simulink model "EiTR2018B (1)"  (R2019b)
settings: Solver=VariableStepAuto  StartTime=0.0  StopTime=600  RelTol=1e-3
values from neighbouring files (symbols this model uses):
  boardingTime = 15    [configFile.m]
  transportTime = 60    [configFile.m]
undefined symbols (not defined in the file or in its folder): m, n
(part 2 of 2)

== stateflow chart EiTR2018B (1)/Person generator two ==
  settings: enableNonTerminalStates=1
  state Hour_24
    state min_0
      state IDLE
        entry:
        lambda = 4;
        dt =60* rand();
        Persons.data=poissrnd(lambda);
      state Wait
      (default) -> Hour_24.min_0.IDLE
      Hour_24.min_0.Wait -> Hour_24.min_0.IDLE : after(dt,sec){send(Persons)}
      Hour_24.min_0.IDLE -> Hour_24.min_0.Wait
    state min_45
      state IDLE
        entry:
        lambda = 4;
        dt =60* rand();
        Persons.data=poissrnd(lambda);
      state Wait
      (default) -> Hour_24.min_45.IDLE : {dt=0;}
      Hour_24.min_45.Wait -> Hour_24.min_45.IDLE : after(dt,sec){send(Persons)}
      Hour_24.min_45.IDLE -> Hour_24.min_45.Wait
    state min_15
      state IDLE
        entry:
        lambda = 4;
        dt =60* rand();
        Persons.data=poissrnd(lambda);
      state Wait
      (default) -> Hour_24.min_15.IDLE : {dt=0;}
      Hour_24.min_15.Wait -> Hour_24.min_15.IDLE : after(dt,sec){send(Persons)}
      Hour_24.min_15.IDLE -> Hour_24.min_15.Wait
    state min_30
      state IDLE
        entry:
        lambda = 4;
        dt =60* rand();
        Persons.data=poissrnd(lambda);
      state Wait
      (default) -> Hour_24.min_30.IDLE : {dt=0;}
      Hour_24.min_30.Wait -> Hour_24.min_30.IDLE : after(dt,sec){send(Persons)}
      Hour_24.min_30.IDLE -> Hour_24.min_30.Wait
    (default) -> Hour_24.min_0
    Hour_24.min_0 -> Hour_24.min_15 : after(60*15,sec)
    Hour_24.min_30 -> Hour_24.min_45 : after(60*15,sec)
    Hour_24.min_15 -> Hour_24.min_30 : after(60*15,sec)
  state Hour_23
    state min_0
      state IDLE
        entry:
        lambda = 4;
        dt =60* rand();
        Persons.data=poissrnd(lambda);
      state Wait
      (default) -> Hour_23.min_0.IDLE
      Hour_23.min_0.Wait -> Hour_23.min_0.IDLE : after(dt,sec){send(Persons)}
      Hour_23.min_0.IDLE -> Hour_23.min_0.Wait
    state min_45
      state IDLE
        entry:
        lambda = 4;
        dt =60* rand();
        Persons.data=poissrnd(lambda);
      state Wait
      (default) -> Hour_23.min_45.IDLE : {dt=0;}
      Hour_23.min_45.Wait -> Hour_23.min_45.IDLE : after(dt,sec){send(Persons)}
      Hour_23.min_45.IDLE -> Hour_23.min_45.Wait
    state min_15
      state IDLE
        entry:
        lambda = 4;
        dt =60* rand();
        Persons.data=poissrnd(lambda);
      state Wait
      (default) -> Hour_23.min_15.IDLE : {dt=0;}
      Hour_23.min_15.Wait -> Hour_23.min_15.IDLE : after(dt,sec){send(Persons)}
      Hour_23.min_15.IDLE -> Hour_23.min_15.Wait
    state min_30
      state IDLE
        entry:
        lambda = 4;
        dt =60* rand();
        Persons.data=poissrnd(lambda);
      state Wait
      (default) -> Hour_23.min_30.IDLE : {dt=0;}
      Hour_23.min_30.Wait -> Hour_23.min_30.IDLE : after(dt,sec){send(Persons)}
      Hour_23.min_30.IDLE -> Hour_23.min_30.Wait
    (default) -> Hour_23.min_0
    Hour_23.min_0 -> Hour_23.min_15 : after(60*15,sec)
    Hour_23.min_30 -> Hour_23.min_45 : after(60*15,sec)
    Hour_23.min_15 -> Hour_23.min_30 : after(60*15,sec)
  state Hour_1
    state min_0
      state IDLE
        entry:
        lambda = 0.5;
        dt =60* rand();
        Persons.data=poissrnd(lambda);
      state Wait
      (default) -> Hour_1.min_0.IDLE
      Hour_1.min_0.Wait -> Hour_1.min_0.IDLE : after(dt,sec){send(Persons)}
      Hour_1.min_0.IDLE -> Hour_1.min_0.Wait
    state min_45
      state IDLE
        entry:
        lambda = 4;
        dt =60* rand();
        Persons.data=poissrnd(lambda);
      state Wait
      (default) -> Hour_1.min_45.IDLE : {dt=0;}
      Hour_1.min_45.Wait -> Hour_1.min_45.IDLE : after(dt,sec){send(Persons)}
      Hour_1.min_45.IDLE -> Hour_1.min_45.Wait
    state min_15
      state IDLE
        entry:
        lambda = 0.3;
        dt =60* rand();
        Persons.data=poissrnd(lambda);
      state Wait
      (default) -> Hour_1.min_15.IDLE : {dt=0;}
      Hour_1.min_15.Wait -> Hour_1.min_15.IDLE : after(dt,sec){send(Persons)}
      Hour_1.min_15.IDLE -> Hour_1.min_15.Wait
    state min_30
      state IDLE
        entry:
        lambda = 4;
        dt =60* rand();
        Persons.data=poissrnd(lambda);
      state Wait
      (default) -> Hour_1.min_30.IDLE : {dt=0;}
      Hour_1.min_30.Wait -> Hour_1.min_30.IDLE : after(dt,sec){send(Persons)}
      Hour_1.min_30.IDLE -> Hour_1.min_30.Wait
    (default) -> Hour_1.min_0
    Hour_1.min_0 -> Hour_1.min_15 : after(60*15,sec)
    Hour_1.min_30 -> Hour_1.min_45 : after(60*15,sec)
    Hour_1.min_15 -> Hour_1.min_30 : after(60*15,sec)
  state Hour_22
    state min_0
      state IDLE
        entry:
        lambda = 4;
        dt =60* rand();
        Persons.data=poissrnd(lambda);
      state Wait
      (default) -> Hour_22.min_0.IDLE
      Hour_22.min_0.Wait -> Hour_22.min_0.IDLE : after(dt,sec){send(Persons)}
      Hour_22.min_0.IDLE -> Hour_22.min_0.Wait
    state min_45
      state IDLE
        entry:
        lambda = 4;
        dt =60* rand();
        Persons.data=poissrnd(lambda);
      state Wait
      (default) -> Hour_22.min_45.IDLE : {dt=0;}
      Hour_22.min_45.Wait -> Hour_22.min_45.IDLE : after(dt,sec){send(Persons)}
      Hour_22.min_45.IDLE -> Hour_22.min_45.Wait
    state min_15
      state IDLE
        entry:
        lambda = 4;
        dt =60* rand();
        Persons.data=poissrnd(lambda);
      state Wait
      (default) -> Hour_22.min_15.IDLE : {dt=0;}
      Hour_22.min_15.Wait -> Hour_22.min_15.IDLE : after(dt,sec){send(Persons)}
      Hour_22.min_15.IDLE -> Hour_22.min_15.Wait
    state min_30
      state IDLE
        entry:
        lambda = 4;
        dt =60* rand();
        Persons.data=poissrnd(lambda);
      state Wait
      (default) -> Hour_22.min_30.IDLE : {dt=0;}
      Hour_22.min_30.Wait -> Hour_22.min_30.IDLE : after(dt,sec){send(Persons)}
      Hour_22.min_30.IDLE -> Hour_22.min_30.Wait
    (default) -> Hour_22.min_0
    Hour_22.min_0 -> Hour_22.min_15 : after(60*15,sec)
    Hour_22.min_30 -> Hour_22.min_45 : after(60*15,sec)
    Hour_22.min_15 -> Hour_22.min_30 : after(60*15,sec)
  state Hour_2
    state min_0
      state IDLE
        entry:
        lambda = 4;
        dt =60* rand();
        Persons.data=poissrnd(lambda);
      state Wait
      (default) -> Hour_2.min_0.IDLE
      Hour_2.min_0.Wait -> Hour_2.min_0.IDLE : after(dt,sec){send(Persons)}
      Hour_2.min_0.IDLE -> Hour_2.min_0.Wait
    state min_45
      state IDLE
        entry:
        lambda = 4;
        dt =60* rand();
        Persons.data=poissrnd(lambda);
      state Wait
      (default) -> Hour_2.min_45.IDLE : {dt=0;}
      Hour_2.min_45.Wait -> Hour_2.min_45.IDLE : after(dt,sec){send(Persons)}
      Hour_2.min_45.IDLE -> Hour_2.min_45.Wait
    state min_15
      state IDLE
        entry:
        lambda = 4;
        dt =60* rand();
        Persons.data=poissrnd(lambda);
      state Wait
      (default) -> Hour_2.min_15.IDLE : {dt=0;}
      Hour_2.min_15.Wait -> Hour_2.min_15.IDLE : after(dt,sec){send(Persons)}
      Hour_2.min_15.IDLE -> Hour_2.min_15.Wait
    state min_30
      state IDLE
        entry:
        lambda = 4;
        dt =60* rand();
        Persons.data=poissrnd(lambda);
      state Wait
      (default) -> Hour_2.min_30.IDLE : {dt=0;}
      Hour_2.min_30.Wait -> Hour_2.min_30.IDLE : after(dt,sec){send(Persons)}
      Hour_2.min_30.IDLE -> Hour_2.min_30.Wait
    (default) -> Hour_2.min_0
    Hour_2.min_0 -> Hour_2.min_15 : after(60*15,sec)
    Hour_2.min_30 -> Hour_2.min_45 : after(60*15,sec)
    Hour_2.min_15 -> Hour_2.min_30 : after(60*15,sec)
  state Hour_21
    state min_0
      state IDLE
        entry:
        lambda = 4;
        dt =60* rand();
        Persons.data=poissrnd(lambda);
      state Wait
      (default) -> Hour_21.min_0.IDLE
      Hour_21.min_0.Wait -> Hour_21.min_0.IDLE : after(dt,sec){send(Persons)}
      Hour_21.min_0.IDLE -> Hour_21.min_0.Wait
    state min_45
      state IDLE
        entry:
        lambda = 4;
        dt =60* rand();
        Persons.data=poissrnd(lambda);
      state Wait
      (default) -> Hour_21.min_45.IDLE : {dt=0;}
      Hour_21.min_45.Wait -> Hour_21.min_45.IDLE : after(dt,sec){send(Persons)}
      Hour_21.min_45.IDLE -> Hour_21.min_45.Wait
    state min_15
      state IDLE
        entry:
        lambda = 4;
        dt =60* rand();
        Persons.data=poissrnd(lambda);
      state Wait
      (default) -> Hour_21.min_15.IDLE : {dt=0;}
      Hour_21.min_15.Wait -> Hour_21.min_15.IDLE : after(dt,sec){send(Persons)}
      Hour_21.min_15.IDLE -> Hour_21.min_15.Wait
    state min_30
      state IDLE
        entry:
        lambda = 4;
        dt =60* rand();
        Persons.data=poissrnd(lambda);
      state Wait
      (default) -> Hour_21.min_30.IDLE : {dt=0;}
      Hour_21.min_30.Wait -> Hour_21.min_30.IDLE : after(dt,sec){send(Persons)}
      Hour_21.min_30.IDLE -> Hour_21.min_30.Wait
    (default) -> Hour_21.min_0
    Hour_21.min_0 -> Hour_21.min_15 : after(60*15,sec)
    Hour_21.min_30 -> Hour_21.min_45 : after(60*15,sec)
    Hour_21.min_15 -> Hour_21.min_30 : after(60*15,sec)
  state Hour_3
    state min_0
      state IDLE
        entry:
        lambda = 4;
        dt =60* rand();
        Persons.data=poissrnd(lambda);
      state Wait
      (default) -> Hour_3.min_0.IDLE
      Hour_3.min_0.Wait -> Hour_3.min_0.IDLE : after(dt,sec){send(Persons)}
      Hour_3.min_0.IDLE -> Hour_3.min_0.Wait
    state min_45
      state IDLE
        entry:
        lambda = 4;
        dt =60* rand();
        Persons.data=poissrnd(lambda);
      state Wait
      (default) -> Hour_3.min_45.IDLE : {dt=0;}
      Hour_3.min_45.Wait -> Hour_3.min_45.IDLE : after(dt,sec){send(Persons)}
      Hour_3.min_45.IDLE -> Hour_3.min_45.Wait
    state min_15
      state IDLE
        entry:
        lambda = 4;
        dt =60* rand();
        Persons.data=poissrnd(lambda);
      state Wait
      (default) -> Hour_3.min_15.IDLE : {dt=0;}
      Hour_3.min_15.Wait -> Hour_3.min_15.IDLE : after(dt,sec){send(Persons)}
      Hour_3.min_15.IDLE -> Hour_3.min_15.Wait
    state min_30
      state IDLE
        entry:
        lambda = 4;
        dt =60* rand();
        Persons.data=poissrnd(lambda);
      state Wait
      (default) -> Hour_3.min_30.IDLE : {dt=0;}
      Hour_3.min_30.Wait -> Hour_3.min_30.IDLE : after(dt,sec){send(Persons)}
      Hour_3.min_30.IDLE -> Hour_3.min_30.Wait
    (default) -> Hour_3.min_0
    Hour_3.min_0 -> Hour_3.min_15 : after(60*15,sec)
    Hour_3.min_30 -> Hour_3.min_45 : after(60*15,sec)
    Hour_3.min_15 -> Hour_3.min_30 : after(60*15,sec)
  state Hour_20
    state min_0
      state IDLE
        entry:
        lambda = 4;
        dt =60* rand();
        Persons.data=poissrnd(lambda);
      state Wait
      (default) -> Hour_20.min_0.IDLE
      Hour_20.min_0.Wait -> Hour_20.min_0.IDLE : after(dt,sec){send(Persons)}
      Hour_20.min_0.IDLE -> Hour_20.min_0.Wait
    state min_45
      state IDLE
        entry:
        lambda = 4;
        dt =60* rand();
        Persons.data=poissrnd(lambda);
      state Wait
      (default) -> Hour_20.min_45.IDLE : {dt=0;}
      Hour_20.min_45.Wait -> Hour_20.min_45.IDLE : after(dt,sec){send(Persons)}
      Hour_20.min_45.IDLE -> Hour_20.min_45.Wait
    state min_15
      state IDLE
        entry:
        lambda = 4;
        dt =60* rand();
        Persons.data=poissrnd(lambda);
      state Wait
      (default) -> Hour_20.min_15.IDLE : {dt=0;}
      Hour_20.min_15.Wait -> Hour_20.min_15.IDLE : after(dt,sec){send(Persons)}
      Hour_20.min_15.IDLE -> Hour_20.min_15.Wait
    state min_30
      state IDLE
        entry:
        lambda = 4;
        dt =60* rand();
        Persons.data=poissrnd(lambda);
      state Wait
      (default) -> Hour_20.min_30.IDLE : {dt=0;}
      Hour_20.min_30.Wait -> Hour_20.min_30.IDLE : after(dt,sec){send(Persons)}
      Hour_20.min_30.IDLE -> Hour_20.min_30.Wait
    (default) -> Hour_20.min_0
    Hour_20.min_0 -> Hour_20.min_15 : after(60*15,sec)
    Hour_20.min_30 -> Hour_20.min_45 : after(60*15,sec)
    Hour_20.min_15 -> Hour_20.min_30 : after(60*15,sec)
  state Hour_4
    state min_0
      state IDLE
        entry:
        lambda = 4;
        dt =60* rand();
        Persons.data=poissrnd(lambda);
      state Wait
      (default) -> Hour_4.min_0.IDLE
      Hour_4.min_0.Wait -> Hour_4.min_0.IDLE : after(dt,sec){send(Persons)}
      Hour_4.min_0.IDLE -> Hour_4.min_0.Wait
    state min_45
      state IDLE
        entry:
        lambda = 4;
        dt =60* rand();
        Persons.data=poissrnd(lambda);
      state Wait
      (default) -> Hour_4.min_45.IDLE : {dt=0;}
      Hour_4.min_45.Wait -> Hour_4.min_45.IDLE : after(dt,sec){send(Persons)}
      Hour_4.min_45.IDLE -> Hour_4.min_45.Wait
    state min_15
      state IDLE
        entry:
        lambda = 4;
        dt =60* rand();
        Persons.data=poissrnd(lambda);
      state Wait
      (default) -> Hour_4.min_15.IDLE : {dt=0;}
      Hour_4.min_15.Wait -> Hour_4.min_15.IDLE : after(dt,sec){send(Persons)}
      Hour_4.min_15.IDLE -> Hour_4.min_15.Wait
    state min_30
      state IDLE
        entry:
        lambda = 4;
        dt =60* rand();
        Persons.data=poissrnd(lambda);
      state Wait
      (default) -> Hour_4.min_30.IDLE : {dt=0;}
      Hour_4.min_30.Wait -> Hour_4.min_30.IDLE : after(dt,sec){send(Persons)}
      Hour_4.min_30.IDLE -> Hour_4.min_30.Wait
    (default) -> Hour_4.min_0
    Hour_4.min_0 -> Hour_4.min_15 : after(60*15,sec)
    Hour_4.min_30 -> Hour_4.min_45 : after(60*15,sec)
    Hour_4.min_15 -> Hour_4.min_30 : after(60*15,sec)
  state Hour_19
    state min_0
      state IDLE
        entry:
        lambda = 4;
        dt =60* rand();
        Persons.data=poissrnd(lambda);
      state Wait
      (default) -> Hour_19.min_0.IDLE
      Hour_19.min_0.Wait -> Hour_19.min_0.IDLE : after(dt,sec){send(Persons)}
      Hour_19.min_0.IDLE -> Hour_19.min_0.Wait
    state min_45
      state IDLE
        entry:
        lambda = 4;
        dt =60* rand();
        Persons.data=poissrnd(lambda);
      state Wait
      (default) -> Hour_19.min_45.IDLE : {dt=0;}
      Hour_19.min_45.Wait -> Hour_19.min_45.IDLE : after(dt,sec){send(Persons)}
      Hour_19.min_45.IDLE -> Hour_19.min_45.Wait
    state min_15
      state IDLE
        entry:
        lambda = 4;
        dt =60* rand();
        Persons.data=poissrnd(lambda);
      state Wait
      (default) -> Hour_19.min_15.IDLE : {dt=0;}
      Hour_19.min_15.Wait -> Hour_19.min_15.IDLE : after(dt,sec){send(Persons)}
      Hour_19.min_15.IDLE -> Hour_19.min_15.Wait
    state min_30
      state IDLE
        entry:
        lambda = 4;
        dt =60* rand();
        Persons.data=poissrnd(lambda);
      state Wait
      (default) -> Hour_19.min_30.IDLE : {dt=0;}
      Hour_19.min_30.Wait -> Hour_19.min_30.IDLE : after(dt,sec){send(Persons)}
      Hour_19.min_30.IDLE -> Hour_19.min_30.Wait
    (default) -> Hour_19.min_0
    Hour_19.min_0 -> Hour_19.min_15 : after(60*15,sec)
    Hour_19.min_30 -> Hour_19.min_45 : after(60*15,sec)
    Hour_19.min_15 -> Hour_19.min_30 : after(60*15,sec)
  state Hour_5
    state min_0
      state IDLE
        entry:
        lambda = 4;
        dt =60* rand();
        Persons.data=poissrnd(lambda);
      state Wait
      (default) -> Hour_5.min_0.IDLE
      Hour_5.min_0.Wait -> Hour_5.min_0.IDLE : after(dt,sec){send(Persons)}
      Hour_5.min_0.IDLE -> Hour_5.min_0.Wait
    state min_45
      state IDLE
        entry:
        lambda = 4;
        dt =60* rand();
        Persons.data=poissrnd(lambda);
      state Wait
      (default) -> Hour_5.min_45.IDLE : {dt=0;}
      Hour_5.min_45.Wait -> Hour_5.min_45.IDLE : after(dt,sec){send(Persons)}
      Hour_5.min_45.IDLE -> Hour_5.min_45.Wait
    state min_15
      state IDLE
        entry:
        lambda = 4;
        dt =60* rand();
        Persons.data=poissrnd(lambda);
      state Wait
      (default) -> Hour_5.min_15.IDLE : {dt=0;}
      Hour_5.min_15.Wait -> Hour_5.min_15.IDLE : after(dt,sec){send(Persons)}
      Hour_5.min_15.IDLE -> Hour_5.min_15.Wait
    state min_30
      state IDLE
        entry:
        lambda = 4;
        dt =60* rand();
        Persons.data=poissrnd(lambda);
      state Wait
      (default) -> Hour_5.min_30.IDLE : {dt=0;}
      Hour_5.min_30.Wait -> Hour_5.min_30.IDLE : after(dt,sec){send(Persons)}
      Hour_5.min_30.IDLE -> Hour_5.min_30.Wait
    (default) -> Hour_5.min_0
    Hour_5.min_0 -> Hour_5.min_15 : after(60*15,sec)
    Hour_5.min_30 -> Hour_5.min_45 : after(60*15,sec)
    Hour_5.min_15 -> Hour_5.min_30 : after(60*15,sec)
  state Hour_18
    state min_0
      state IDLE
        entry:
        lambda = 4;
        dt =60* rand();
        Persons.data=poissrnd(lambda);
      state Wait
      (default) -> Hour_18.min_0.IDLE
      Hour_18.min_0.Wait -> Hour_18.min_0.IDLE : after(dt,sec){send(Persons)}
      Hour_18.min_0.IDLE -> Hour_18.min_0.Wait
    state min_45
      state IDLE
        entry:
        lambda = 4;
        dt =60* rand();
        Persons.data=poissrnd(lambda);
      state Wait
      (default) -> Hour_18.min_45.IDLE : {dt=0;}
      Hour_18.min_45.Wait -> Hour_18.min_45.IDLE : after(dt,sec){send(Persons)}
      Hour_18.min_45.IDLE -> Hour_18.min_45.Wait
    state min_15
      state IDLE
        entry:
        lambda = 4;
        dt =60* rand();
        Persons.data=poissrnd(lambda);
      state Wait
      (default) -> Hour_18.min_15.IDLE : {dt=0;}
      Hour_18.min_15.Wait -> Hour_18.min_15.IDLE : after(dt,sec){send(Persons)}
      Hour_18.min_15.IDLE -> Hour_18.min_15.Wait
    state min_30
      state IDLE
        entry:
        lambda = 4;
        dt =60* rand();
        Persons.data=poissrnd(lambda);
      state Wait
      (default) -> Hour_18.min_30.IDLE : {dt=0;}
      Hour_18.min_30.Wait -> Hour_18.min_30.IDLE : after(dt,sec){send(Persons)}
      Hour_18.min_30.IDLE -> Hour_18.min_30.Wait
    (default) -> Hour_18.min_0
    Hour_18.min_0 -> Hour_18.min_15 : after(60*15,sec)
    Hour_18.min_30 -> Hour_18.min_45 : after(60*15,sec)
    Hour_18.min_15 -> Hour_18.min_30 : after(60*15,sec)
  state Hour_6
    state min_0
      state IDLE
        entry:
        lambda = 4;
        dt =60* rand();
        Persons.data=poissrnd(lambda);
      state Wait
      (default) -> Hour_6.min_0.IDLE
      Hour_6.min_0.Wait -> Hour_6.min_0.IDLE : after(dt,sec){send(Persons)}
      Hour_6.min_0.IDLE -> Hour_6.min_0.Wait
    state min_45
      state IDLE
        entry:
        lambda = 4;
        dt =60* rand();
        Persons.data=poissrnd(lambda);
      state Wait
      (default) -> Hour_6.min_45.IDLE : {dt=0;}
      Hour_6.min_45.Wait -> Hour_6.min_45.IDLE : after(dt,sec){send(Persons)}
      Hour_6.min_45.IDLE -> Hour_6.min_45.Wait
    state min_15
      state IDLE
        entry:
        lambda = 4;
        dt =60* rand();
        Persons.data=poissrnd(lambda);
      state Wait
      (default) -> Hour_6.min_15.IDLE : {dt=0;}
      Hour_6.min_15.Wait -> Hour_6.min_15.IDLE : after(dt,sec){send(Persons)}
      Hour_6.min_15.IDLE -> Hour_6.min_15.Wait
    state min_30
      state IDLE
        entry:
        lambda = 4;
        dt =60* rand();
        Persons.data=poissrnd(lambda);
      state Wait
      (default) -> Hour_6.min_30.IDLE : {dt=0;}
      Hour_6.min_30.Wait -> Hour_6.min_30.IDLE : after(dt,sec){send(Persons)}
      Hour_6.min_30.IDLE -> Hour_6.min_30.Wait
    (default) -> Hour_6.min_0
    Hour_6.min_0 -> Hour_6.min_15 : after(60*15,sec)
    Hour_6.min_30 -> Hour_6.min_45 : after(60*15,sec)
    Hour_6.min_15 -> Hour_6.min_30 : after(60*15,sec)
  state Hour_17
    state min_0
      state IDLE
        entry:
        lambda = 4;
        dt =60* rand();
        Persons.data=poissrnd(lambda);
      state Wait
      (default) -> Hour_17.min_0.IDLE
      Hour_17.min_0.Wait -> Hour_17.min_0.IDLE : after(dt,sec){send(Persons)}
      Hour_17.min_0.IDLE -> Hour_17.min_0.Wait
    state min_45
      state IDLE
        entry:
        lambda = 4;
        dt =60* rand();
        Persons.data=poissrnd(lambda);
      state Wait
      (default) -> Hour_17.min_45.IDLE : {dt=0;}
      Hour_17.min_45.Wait -> Hour_17.min_45.IDLE : after(dt,sec){send(Persons)}
      Hour_17.min_45.IDLE -> Hour_17.min_45.Wait
    state min_15
      state IDLE
        entry:
        lambda = 4;
        dt =60* rand();
        Persons.data=poissrnd(lambda);
      state Wait
      (default) -> Hour_17.min_15.IDLE : {dt=0;}
      Hour_17.min_15.Wait -> Hour_17.min_15.IDLE : after(dt,sec){send(Persons)}
      Hour_17.min_15.IDLE -> Hour_17.min_15.Wait
    state min_30
      state IDLE
        entry:
        lambda = 4;
        dt =60* rand();
        Persons.data=poissrnd(lambda);
      state Wait
      (default) -> Hour_17.min_30.IDLE : {dt=0;}
      Hour_17.min_30.Wait -> Hour_17.min_30.IDLE : after(dt,sec){send(Persons)}
      Hour_17.min_30.IDLE -> Hour_17.min_30.Wait
    (default) -> Hour_17.min_0
    Hour_17.min_0 -> Hour_17.min_15 : after(60*15,sec)
    Hour_17.min_30 -> Hour_17.min_45 : after(60*15,sec)
    Hour_17.min_15 -> Hour_17.min_30 : after(60*15,sec)
  state Hour_7
    state min_0
      state IDLE
        entry:
        lambda = 4;
        dt =60* rand();
        Persons.data=poissrnd(lambda);
      state Wait
      (default) -> Hour_7.min_0.IDLE
      Hour_7.min_0.Wait -> Hour_7.min_0.IDLE : after(dt,sec){send(Persons)}
      Hour_7.min_0.IDLE -> Hour_7.min_0.Wait
    state min_45
      state IDLE
        entry:
        lambda = 4;
        dt =60* rand();
        Persons.data=poissrnd(lambda);
      state Wait
      (default) -> Hour_7.min_45.IDLE : {dt=0;}
      Hour_7.min_45.Wait -> Hour_7.min_45.IDLE : after(dt,sec){send(Persons)}
      Hour_7.min_45.IDLE -> Hour_7.min_45.Wait
    state min_15
      state IDLE
        entry:
        lambda = 4;
        dt =60* rand();
        Persons.data=poissrnd(lambda);
      state Wait
      (default) -> Hour_7.min_15.IDLE : {dt=0;}
      Hour_7.min_15.Wait -> Hour_7.min_15.IDLE : after(dt,sec){send(Persons)}
      Hour_7.min_15.IDLE -> Hour_7.min_15.Wait
    state min_30
      state IDLE
        entry:
        lambda = 4;
        dt =60* rand();
        Persons.data=poissrnd(lambda);
      state Wait
      (default) -> Hour_7.min_30.IDLE : {dt=0;}
      Hour_7.min_30.Wait -> Hour_7.min_30.IDLE : after(dt,sec){send(Persons)}
      Hour_7.min_30.IDLE -> Hour_7.min_30.Wait
    (default) -> Hour_7.min_0
    Hour_7.min_0 -> Hour_7.min_15 : after(60*15,sec)
    Hour_7.min_30 -> Hour_7.min_45 : after(60*15,sec)
    Hour_7.min_15 -> Hour_7.min_30 : after(60*15,sec)
  state Hour_16
    state min_0
      state IDLE
        entry:
        lambda = 4;
        dt =60* rand();
        Persons.data=poissrnd(lambda);
      state Wait
      (default) -> Hour_16.min_0.IDLE
      Hour_16.min_0.Wait -> Hour_16.min_0.IDLE : after(dt,sec){send(Persons)}
      Hour_16.min_0.IDLE -> Hour_16.min_0.Wait
    state min_45
      state IDLE
        entry:
        lambda = 4;
        dt =60* rand();
        Persons.data=poissrnd(lambda);
      state Wait
      (default) -> Hour_16.min_45.IDLE : {dt=0;}
      Hour_16.min_45.Wait -> Hour_16.min_45.IDLE : after(dt,sec){send(Persons)}
      Hour_16.min_45.IDLE -> Hour_16.min_45.Wait
    state min_15
      state IDLE
        entry:
        lambda = 4;
        dt =60* rand();
        Persons.data=poissrnd(lambda);
      state Wait
      (default) -> Hour_16.min_15.IDLE : {dt=0;}
      Hour_16.min_15.Wait -> Hour_16.min_15.IDLE : after(dt,sec){send(Persons)}
      Hour_16.min_15.IDLE -> Hour_16.min_15.Wait
    state min_30
      state IDLE
        entry:
        lambda = 4;
        dt =60* rand();
        Persons.data=poissrnd(lambda);
      state Wait
      (default) -> Hour_16.min_30.IDLE : {dt=0;}
      Hour_16.min_30.Wait -> Hour_16.min_30.IDLE : after(dt,sec){send(Persons)}
      Hour_16.min_30.IDLE -> Hour_16.min_30.Wait
    (default) -> Hour_16.min_0
    Hour_16.min_0 -> Hour_16.min_15 : after(60*15,sec)
    Hour_16.min_30 -> Hour_16.min_45 : after(60*15,sec)
    Hour_16.min_15 -> Hour_16.min_30 : after(60*15,sec)
  state Hour_8
    state min_0
      state IDLE
        entry:
        lambda = 4;
        dt =60* rand();
        Persons.data=poissrnd(lambda);
      state Wait
      (default) -> Hour_8.min_0.IDLE
      Hour_8.min_0.Wait -> Hour_8.min_0.IDLE : after(dt,sec){send(Persons)}
      Hour_8.min_0.IDLE -> Hour_8.min_0.Wait
    state min_45
      state IDLE
        entry:
        lambda = 4;
        dt =60* rand();
        Persons.data=poissrnd(lambda);
      state Wait
      (default) -> Hour_8.min_45.IDLE : {dt=0;}
      Hour_8.min_45.Wait -> Hour_8.min_45.IDLE : after(dt,sec){send(Persons)}
      Hour_8.min_45.IDLE -> Hour_8.min_45.Wait
    state min_15
      state IDLE
        entry:
        lambda = 4;
        dt =60* rand();
        Persons.data=poissrnd(lambda);
      state Wait
      (default) -> Hour_8.min_15.IDLE : {dt=0;}
      Hour_8.min_15.Wait -> Hour_8.min_15.IDLE : after(dt,sec){send(Persons)}
      Hour_8.min_15.IDLE -> Hour_8.min_15.Wait
    state min_30
      state IDLE
        entry:
        lambda = 4;
        dt =60* rand();
        Persons.data=poissrnd(lambda);
      state Wait
      (default) -> Hour_8.min_30.IDLE : {dt=0;}
      Hour_8.min_30.Wait -> Hour_8.min_30.IDLE : after(dt,sec){send(Persons)}
      Hour_8.min_30.IDLE -> Hour_8.min_30.Wait
    (default) -> Hour_8.min_0
    Hour_8.min_0 -> Hour_8.min_15 : after(60*15,sec)
    Hour_8.min_30 -> Hour_8.min_45 : after(60*15,sec)
    Hour_8.min_15 -> Hour_8.min_30 : after(60*15,sec)
  state Hour_15
    state min_0
      state IDLE
        entry:
        lambda = 4;
        dt =60* rand();
        Persons.data=poissrnd(lambda);
      state Wait
      (default) -> Hour_15.min_0.IDLE
      Hour_15.min_0.Wait -> Hour_15.min_0.IDLE : after(dt,sec){send(Persons)}
      Hour_15.min_0.IDLE -> Hour_15.min_0.Wait
    state min_45
      state IDLE
        entry:
        lambda = 4;
        dt =60* rand();
        Persons.data=poissrnd(lambda);
      state Wait
      (default) -> Hour_15.min_45.IDLE : {dt=0;}
      Hour_15.min_45.Wait -> Hour_15.min_45.IDLE : after(dt,sec){send(Persons)}
      Hour_15.min_45.IDLE -> Hour_15.min_45.Wait
    state min_15
      state IDLE
        entry:
        lambda = 4;
        dt =60* rand();
        Persons.data=poissrnd(lambda);
      state Wait
      (default) -> Hour_15.min_15.IDLE : {dt=0;}
      Hour_15.min_15.Wait -> Hour_15.min_15.IDLE : after(dt,sec){send(Persons)}
      Hour_15.min_15.IDLE -> Hour_15.min_15.Wait
    state min_30
      state IDLE
        entry:
        lambda = 4;
        dt =60* rand();
        Persons.data=poissrnd(lambda);
      state Wait
      (default) -> Hour_15.min_30.IDLE : {dt=0;}
      Hour_15.min_30.Wait -> Hour_15.min_30.IDLE : after(dt,sec){send(Persons)}
      Hour_15.min_30.IDLE -> Hour_15.min_30.Wait
    (default) -> Hour_15.min_0
    Hour_15.min_0 -> Hour_15.min_15 : after(60*15,sec)
    Hour_15.min_30 -> Hour_15.min_45 : after(60*15,sec)
    Hour_15.min_15 -> Hour_15.min_30 : after(60*15,sec)
  state Hour_14
    state min_0
      state IDLE
        entry:
        lambda = 4;
        dt =60* rand();
        Persons.data=poissrnd(lambda);
      state Wait
      (default) -> Hour_14.min_0.IDLE
      Hour_14.min_0.Wait -> Hour_14.min_0.IDLE : after(dt,sec){send(Persons)}
      Hour_14.min_0.IDLE -> Hour_14.min_0.Wait
    state min_45
      state IDLE
        entry:
        lambda = 4;
        dt =60* rand();
        Persons.data=poissrnd(lambda);
      state Wait
      (default) -> Hour_14.min_45.IDLE : {dt=0;}
      Hour_14.min_45.Wait -> Hour_14.min_45.IDLE : after(dt,sec){send(Persons)}
      Hour_14.min_45.IDLE -> Hour_14.min_45.Wait
    state min_15
      state IDLE
        entry:
        lambda = 4;
        dt =60* rand();
        Persons.data=poissrnd(lambda);
      state Wait
      (default) -> Hour_14.min_15.IDLE : {dt=0;}
      Hour_14.min_15.Wait -> Hour_14.min_15.IDLE : after(dt,sec){send(Persons)}
      Hour_14.min_15.IDLE -> Hour_14.min_15.Wait
    state min_30
      state IDLE
        entry:
        lambda = 4;
        dt =60* rand();
        Persons.data=poissrnd(lambda);
      state Wait
      (default) -> Hour_14.min_30.IDLE : {dt=0;}
      Hour_14.min_30.Wait -> Hour_14.min_30.IDLE : after(dt,sec){send(Persons)}
      Hour_14.min_30.IDLE -> Hour_14.min_30.Wait
    (default) -> Hour_14.min_0
    Hour_14.min_0 -> Hour_14.min_15 : after(60*15,sec)
    Hour_14.min_30 -> Hour_14.min_45 : after(60*15,sec)
    Hour_14.min_15 -> Hour_14.min_30 : after(60*15,sec)
  state Hour_9
    state min_0
      state IDLE
        entry:
        lambda = 4;
        dt =60* rand();
        Persons.data=poissrnd(lambda);
      state Wait
      (default) -> Hour_9.min_0.IDLE
      Hour_9.min_0.Wait -> Hour_9.min_0.IDLE : after(dt,sec){send(Persons)}
      Hour_9.min_0.IDLE -> Hour_9.min_0.Wait
    state min_45
      state IDLE
        entry:
        lambda = 4;
        dt =60* rand();
        Persons.data=poissrnd(lambda);
      state Wait
      (default) -> Hour_9.min_45.IDLE : {dt=0;}
      Hour_9.min_45.Wait -> Hour_9.min_45.IDLE : after(dt,sec){send(Persons)}
      Hour_9.min_45.IDLE -> Hour_9.min_45.Wait
    state min_15
      state IDLE
        entry:
        lambda = 4;
        dt =60* rand();
        Persons.data=poissrnd(lambda);
      state Wait
      (default) -> Hour_9.min_15.IDLE : {dt=0;}
      Hour_9.min_15.Wait -> Hour_9.min_15.IDLE : after(dt,sec){send(Persons)}
      Hour_9.min_15.IDLE -> Hour_9.min_15.Wait
    state min_30
      state IDLE
        entry:
        lambda = 4;
        dt =60* rand();
        Persons.data=poissrnd(lambda);
      state Wait
      (default) -> Hour_9.min_30.IDLE : {dt=0;}
      Hour_9.min_30.Wait -> Hour_9.min_30.IDLE : after(dt,sec){send(Persons)}
      Hour_9.min_30.IDLE -> Hour_9.min_30.Wait
    (default) -> Hour_9.min_0
    Hour_9.min_0 -> Hour_9.min_15 : after(60*15,sec)
    Hour_9.min_30 -> Hour_9.min_45 : after(60*15,sec)
    Hour_9.min_15 -> Hour_9.min_30 : after(60*15,sec)
  state Hour_10
    state min_0
      state IDLE
        entry:
        lambda = 4;
        dt =60* rand();
        Persons.data=poissrnd(lambda);
      state Wait
      (default) -> Hour_10.min_0.IDLE
      Hour_10.min_0.Wait -> Hour_10.min_0.IDLE : after(dt,sec){send(Persons)}
      Hour_10.min_0.IDLE -> Hour_10.min_0.Wait
    state min_45
      state IDLE
        entry:
        lambda = 4;
        dt =60* rand();
        Persons.data=poissrnd(lambda);
      state Wait
      (default) -> Hour_10.min_45.IDLE : {dt=0;}
      Hour_10.min_45.Wait -> Hour_10.min_45.IDLE : after(dt,sec){send(Persons)}
      Hour_10.min_45.IDLE -> Hour_10.min_45.Wait
    state min_15
      state IDLE
        entry:
        lambda = 4;
        dt =60* rand();
        Persons.data=poissrnd(lambda);
      state Wait
      (default) -> Hour_10.min_15.IDLE : {dt=0;}
      Hour_10.min_15.Wait -> Hour_10.min_15.IDLE : after(dt,sec){send(Persons)}
      Hour_10.min_15.IDLE -> Hour_10.min_15.Wait
    state min_30
      state IDLE
        entry:
        lambda = 4;
        dt =60* rand();
        Persons.data=poissrnd(lambda);
      state Wait
      (default) -> Hour_10.min_30.IDLE : {dt=0;}
      Hour_10.min_30.Wait -> Hour_10.min_30.IDLE : after(dt,sec){send(Persons)}
      Hour_10.min_30.IDLE -> Hour_10.min_30.Wait
    (default) -> Hour_10.min_0
    Hour_10.min_0 -> Hour_10.min_15 : after(60*15,sec)
    Hour_10.min_30 -> Hour_10.min_45 : after(60*15,sec)
    Hour_10.min_15 -> Hour_10.min_30 : after(60*15,sec)
  state Hour_13
    state min_0
      state IDLE
        entry:
        lambda = 4;
        dt =60* rand();
        Persons.data=poissrnd(lambda);
      state Wait
      (default) -> Hour_13.min_0.IDLE
      Hour_13.min_0.Wait -> Hour_13.min_0.IDLE : after(dt,sec){send(Persons)}
      Hour_13.min_0.IDLE -> Hour_13.min_0.Wait
    state min_45
      state IDLE
        entry:
        lambda = 4;
        dt =60* rand();
        Persons.data=poissrnd(lambda);
      state Wait
      (default) -> Hour_13.min_45.IDLE : {dt=0;}
      Hour_13.min_45.Wait -> Hour_13.min_45.IDLE : after(dt,sec){send(Persons)}
      Hour_13.min_45.IDLE -> Hour_13.min_45.Wait
    state min_15
      state IDLE
        entry:
        lambda = 4;
        dt =60* rand();
        Persons.data=poissrnd(lambda);
      state Wait
      (default) -> Hour_13.min_15.IDLE : {dt=0;}
      Hour_13.min_15.Wait -> Hour_13.min_15.IDLE : after(dt,sec){send(Persons)}
      Hour_13.min_15.IDLE -> Hour_13.min_15.Wait
    state min_30
      state IDLE
        entry:
        lambda = 4;
        dt =60* rand();
        Persons.data=poissrnd(lambda);
      state Wait
      (default) -> Hour_13.min_30.IDLE : {dt=0;}
      Hour_13.min_30.Wait -> Hour_13.min_30.IDLE : after(dt,sec){send(Persons)}
      Hour_13.min_30.IDLE -> Hour_13.min_30.Wait
    (default) -> Hour_13.min_0
    Hour_13.min_0 -> Hour_13.min_15 : after(60*15,sec)
    Hour_13.min_30 -> Hour_13.min_45 : after(60*15,sec)
    Hour_13.min_15 -> Hour_13.min_30 : after(60*15,sec)
  state Hour_11
    state min_0
      state IDLE
        entry:
        lambda = 4;
        dt =60* rand();
        Persons.data=poissrnd(lambda);
      state Wait
      (default) -> Hour_11.min_0.IDLE
      Hour_11.min_0.Wait -> Hour_11.min_0.IDLE : after(dt,sec){send(Persons)}
      Hour_11.min_0.IDLE -> Hour_11.min_0.Wait
    state min_45
      state IDLE
        entry:
        lambda = 4;
        dt =60* rand();
        Persons.data=poissrnd(lambda);
      state Wait
      (default) -> Hour_11.min_45.IDLE : {dt=0;}
      Hour_11.min_45.Wait -> Hour_11.min_45.IDLE : after(dt,sec){send(Persons)}
      Hour_11.min_45.IDLE -> Hour_11.min_45.Wait
    state min_15
      state IDLE
        entry:
        lambda = 4;
        dt =60* rand();
        Persons.data=poissrnd(lambda);
      state Wait
      (default) -> Hour_11.min_15.IDLE : {dt=0;}
      Hour_11.min_15.Wait -> Hour_11.min_15.IDLE : after(dt,sec){send(Persons)}
      Hour_11.min_15.IDLE -> Hour_11.min_15.Wait
    state min_30
      state IDLE
        entry:
        lambda = 4;
        dt =60* rand();
        Persons.data=poissrnd(lambda);
      state Wait
      (default) -> Hour_11.min_30.IDLE : {dt=0;}
      Hour_11.min_30.Wait -> Hour_11.min_30.IDLE : after(dt,sec){send(Persons)}
      Hour_11.min_30.IDLE -> Hour_11.min_30.Wait
    (default) -> Hour_11.min_0
    Hour_11.min_0 -> Hour_11.min_15 : after(60*15,sec)
    Hour_11.min_30 -> Hour_11.min_45 : after(60*15,sec)
    Hour_11.min_15 -> Hour_11.min_30 : after(60*15,sec)
  state Hour_12
    state min_0
      state IDLE
        entry:
        lambda = 4;
        dt =60* rand();
        Persons.data=poissrnd(lambda);
      state Wait
      (default) -> Hour_12.min_0.IDLE
      Hour_12.min_0.Wait -> Hour_12.min_0.IDLE : after(dt,sec){send(Persons)}
      Hour_12.min_0.IDLE -> Hour_12.min_0.Wait
    state min_45
      state IDLE
        entry:
        lambda = 4;
        dt =60* rand();
        Persons.data=poissrnd(lambda);
      state Wait
      (default) -> Hour_12.min_45.IDLE : {dt=0;}
      Hour_12.min_45.Wait -> Hour_12.min_45.IDLE : after(dt,sec){send(Persons)}
      Hour_12.min_45.IDLE -> Hour_12.min_45.Wait
    state min_15
      state IDLE
        entry:
        lambda = 4;
        dt =60* rand();
        Persons.data=poissrnd(lambda);
      state Wait
      (default) -> Hour_12.min_15.IDLE : {dt=0;}
      Hour_12.min_15.Wait -> Hour_12.min_15.IDLE : after(dt,sec){send(Persons)}
      Hour_12.min_15.IDLE -> Hour_12.min_15.Wait
    state min_30
      state IDLE
        entry:
        lambda = 4;
        dt =60* rand();
        Persons.data=poissrnd(lambda);
      state Wait
      (default) -> Hour_12.min_30.IDLE : {dt=0;}
      Hour_12.min_30.Wait -> Hour_12.min_30.IDLE : after(dt,sec){send(Persons)}
      Hour_12.min_30.IDLE -> Hour_12.min_30.Wait
    (default) -> Hour_12.min_0
    Hour_12.min_0 -> Hour_12.min_15 : after(60*15,sec)
    Hour_12.min_30 -> Hour_12.min_45 : after(60*15,sec)
    Hour_12.min_15 -> Hour_12.min_30 : after(60*15,sec)
  Hour_24 -> Hour_1 : after(60*60,sec)
  Hour_23 -> Hour_24 : after(60*60,sec)
  Hour_22 -> Hour_23 : after(60*60,sec)
  (default) -> Hour_1 : {
      |  lambda=0;
      |  dt=0;
      |
      | }
  Hour_1 -> Hour_2 : after(60*60,sec)
  Hour_21 -> Hour_22 : after(60*60,sec)
  Hour_2 -> Hour_3 : after(60*60,sec)
  Hour_20 -> Hour_21 : after(60*60,sec)
  Hour_3 -> Hour_4 : after(60*60,sec)
  Hour_19 -> Hour_20 : after(60*60,sec)
  Hour_4 -> Hour_5 : after(60*60,sec)
  Hour_18 -> Hour_19 : after(60*60,sec)
  Hour_5 -> Hour_6 : after(60*60,sec)
  Hour_17 -> Hour_18 : after(60*60,sec)
  Hour_6 -> Hour_7 : after(60*60,sec)
  Hour_16 -> Hour_17 : after(60*60,sec)
  Hour_7 -> Hour_8 : after(60*60,sec)
  Hour_15 -> Hour_16 : after(60*60,sec)
  Hour_8 -> Hour_9 : after(60*60,sec)
  Hour_14 -> Hour_15 : after(60*60,sec)
  Hour_13 -> Hour_14 : after(60*60,sec)
  Hour_9 -> Hour_10 : after(60*60,sec)
  Hour_10 -> Hour_11 : after(60*60,sec)
  Hour_12 -> Hour_13 : after(60*60,sec)
  Hour_11 -> Hour_12 : after(60*60,sec)
  data: Persons output; dt local; lambda local

== stateflow chart EiTR2018B (1)/Control system boat with boarding ==
  settings: enableNonTerminalStates=1
  state ControlSystemBoat [group]
    state UnboardingQuayOne
      entry:
      cmdBoardingQuayOne.data = 1;
      send(cmdBoardingQuayOne);
    state MoveBoatOne
      entry:
      MoveBoatOne.data=1;
      send(MoveBoatOne);
    state BoardingQuayOne
      entry:
      cmdBoardingQuayOne.data=1;
      send(cmdBoardingQuayOne);
    state UnboardingQuayTwo
      entry:
      cmdBoardingQuayTwo.data=1;
      send(cmdBoardingQuayTwo);
    state BoardingQuayTwo
      entry:
      cmdBoardingQuayTwo.data=1;
      send(cmdBoardingQuayTwo);
    state MoveBoatQuayTwo
      entry:
      MoveBoatTwo.data=1;
      send(MoveBoatTwo);
    (default) -> BoardingQuayOne : {
        |  boardingTime=BoardingTime;
        |  transportTime=TransportTime;
        | }
    MoveBoatOne -> UnboardingQuayOne : after(transportTime,sec){MoveBoatOne.data=0; send(MoveBoatOne)}
    BoardingQuayOne -> MoveBoatOne : after(boardingTime,sec){cmdBoardingQuayOne.data=0; send(cmdBoardingQuayOne)}
    UnboardingQuayTwo -> BoardingQuayOne : after(boardingTime,sec)
    UnboardingQuayOne -> BoardingQuayTwo : after(boardingTime,sec)
    MoveBoatQuayTwo -> UnboardingQuayTwo : after(transportTime,sec){MoveBoatTwo.data=0; send(MoveBoatTwo)}
    BoardingQuayTwo -> MoveBoatQuayTwo : after(boardingTime,sec){cmdBoardingQuayTwo.data=0; send(cmdBoardingQuayTwo)}
  data: MoveBoatOne output; TransportTime input; transportTime local; cmdBoardingQuayOne output; MoveBoatTwo output; cmdBoardingQuayTwo output; boardingTime local; BoardingTime input
